simulink model "lab3_zq"  (R2018b)
settings: Solver=VariableStepAuto  StartTime=0.0  StopTime=t_max  MaxStep=0.1  RelTol=1e-3
undefined symbols (not defined in the file): Lo, Lrz, Mo, Mrz, T, t0, y0
settings Model: Creator=lev  LastModifiedBy=lev

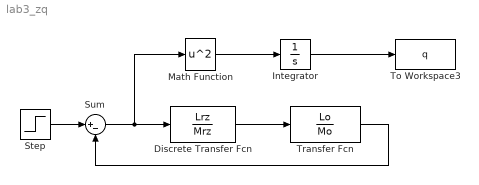
== system lab3_zq ==
  Discrete Transfer Fcn : DiscreteTransferFcn  Numerator=Lrz  Denominator=Mrz  SampleTime=T
  Integrator : Integrator
  Math Function : Math  Operator=square  SaturateOnIntegerOverflow=on
  Step : Step  Time=t0  After=y0  SampleTime=0
  Sum : Sum  Inputs=|+-
  To Workspace3 : ToWorkspace  VariableName=q  SampleTime=-1
      settings: MaxDataPoints=1
  Transfer Fcn : TransferFcn  Numerator=Lo  Denominator=Mo
  wires:
  Transfer Fcn/1 -> Sum/2
  Sum/1 -> Discrete Transfer Fcn/1, Math Function/1
  Step/1 -> Sum/1
  Math Function/1 -> Integrator/1
  Integrator/1 -> To Workspace3/1
  Discrete Transfer Fcn/1 -> Transfer Fcn/1
